simulink model "kfgpPrediction_th"  (R2020a)
settings: Solver=VariableStepAuto  StartTime=0.0  StopTime=10.0  RelTol=1e-3
libraries: kfgpPrediction x1
settings Model: Creator=Ayaz  LastModifiedBy=Ayaz

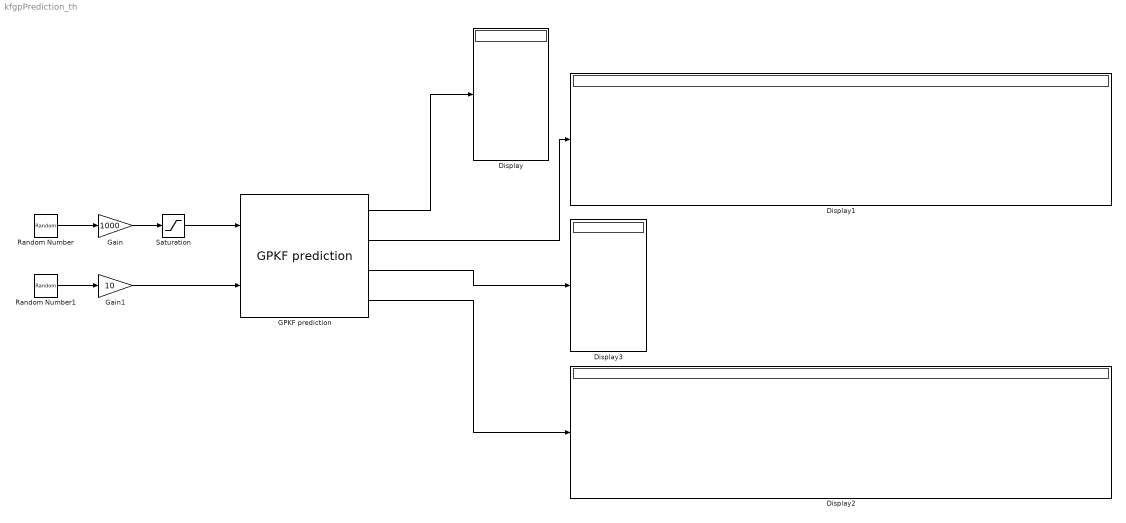
== system kfgpPrediction_th ==
  Display{,1..3} (4 alike) : Display
  GPKF prediction : kfgpPrediction/GPKF prediction  gpkfTimeStep=1  timeScale=22*60  spatialScale=220  covAmp=1  xMeasure=100:100:1000  noiseVar=0.1  hTau='exponential'  powerLawParams=[3.77 0.14]
  Gain : Gain  Gain=1000
  Gain1 : Gain  Gain=10
  Random Number : RandomNumber  SampleTime=0.01
  Random Number1 : RandomNumber  SampleTime=0.01
  Saturation : Saturate  UpperLimit=1000  LowerLimit=100
  wires:
  Gain/1 -> Saturation/1
  Random Number/1 -> Gain/1
  Saturation/1 -> GPKF prediction/1
  Random Number1/1 -> Gain1/1
  Gain1/1 -> GPKF prediction/2
  GPKF prediction/1 -> Display/1
  GPKF prediction/2 -> Display1/1
  GPKF prediction/3 -> Display3/1
  GPKF prediction/4 -> Display2/1
